simulink model "ESP32_AnalogSensor"  (R2025b)
settings: Solver=VariableStepAuto  StartTime=0.0  StopTime=10.0  RelTol=1e-3
libraries: arduinolib x2, simulink x1
settings Model: Creator=anifa  LastModifiedBy=anifa

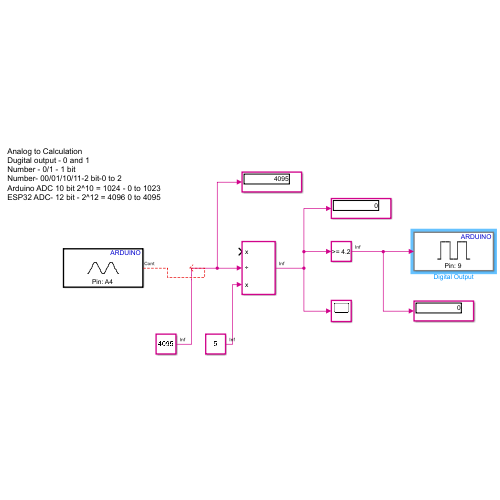
[thumbnail: Simulink's stored preview of the top-level diagram]
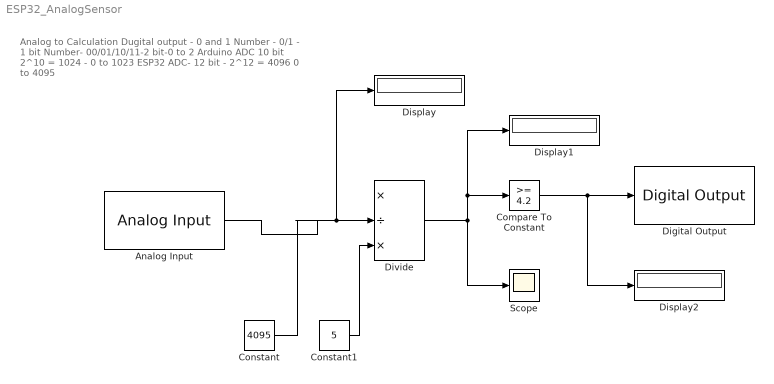
== system ESP32_AnalogSensor ==
  note: Analog to Calculation
      | Dugital output - 0 and 1
      | Number - 0/1 - 1 bit
      | Number- 00/01/10/11-2 bit-0 to 2
      | Arduino ADC 10 bit 2^10 = 1024 - 0 to 1023
      | ESP32 ADC- 12 bit - 2^12 = 4096 0 to 4095
  Analog Input : arduinolib/Analog Input  pinNumber=4  ReadResultsOnly=off  ConversionTriggerSource=Software  ExternalTriggerType=uint32( 0 )  OutputDataType=uint16  EnableConversionCompleteNotify=off  EnableOuputStatus=off  SampleTime=-1  blockPlatform=arduino
  Compare To Constant : simulink/Logic and Bit Operations/Compare To Constant  relop=>=  const=4.2  OutDataTypeStr=boolean
  Constant : Constant  Value=4095
  Constant1 : Constant  Value=5
  Digital Output : arduinolib/Digital Output  pinNumber=9  Direction=output  blockPlatform=arduino
  Display : Display
  Display1 : Display
  Display2 : Display
  Divide : Product  Inputs=*/*
  Scope : Scope
  wires:
  Constant/1 -> Display/1, Divide/2
  Constant1/1 -> Divide/3
  Analog Input/1 -> ?
  Divide/1 -> Display1/1, Compare To Constant/1, Scope/1
  Compare To Constant/1 -> Digital Output/1, Display2/1
